simulink model "d_1_dc_motor"  (R2014b)
settings: Solver=ode45  StartTime=0.0  StopTime=10  RelTol=1e-3
values from neighbouring files (symbols this model uses):
  Bm = 0.01    [d_1_dc_motor_parameter.m]    (also in d_2_draw_wt_theta_real.m; d_2_draw_wt_theta_tf.m; d_4_dc_motor_bar_parameter.m; plot.m)
  Jm = 0.000052    (= 5.2e-05)    [d_1_dc_motor_parameter.m]    (also in d_2_draw_wt_theta_real.m; d_2_draw_wt_theta_tf.m; d_4_dc_motor_bar_parameter.m; plot.m)
  Ke = 0.235    [d_1_dc_motor_parameter.m]    (also in d_2_draw_wt_theta_real.m; d_2_draw_wt_theta_tf.m; d_4_dc_motor_bar_parameter.m; plot.m)
  Kt = 0.235    [d_1_dc_motor_parameter.m]    (also in d_2_draw_wt_theta_real.m; d_2_draw_wt_theta_tf.m; d_4_dc_motor_bar_parameter.m; plot.m)
  La = 0.23    [d_1_dc_motor_parameter.m]    (also in d_2_draw_wt_theta_real.m; d_2_draw_wt_theta_tf.m; d_4_dc_motor_bar_parameter.m; plot.m)
  Ra = 2    [d_1_dc_motor_parameter.m]    (also in d_2_draw_wt_theta_real.m; d_2_draw_wt_theta_tf.m; d_4_dc_motor_bar_parameter.m; plot.m)
  Vlimit = 24    [d_1_dc_motor_parameter.m]
libraries: simulink x3
settings Model: Creator=Admin  LastModifiedBy=Admin

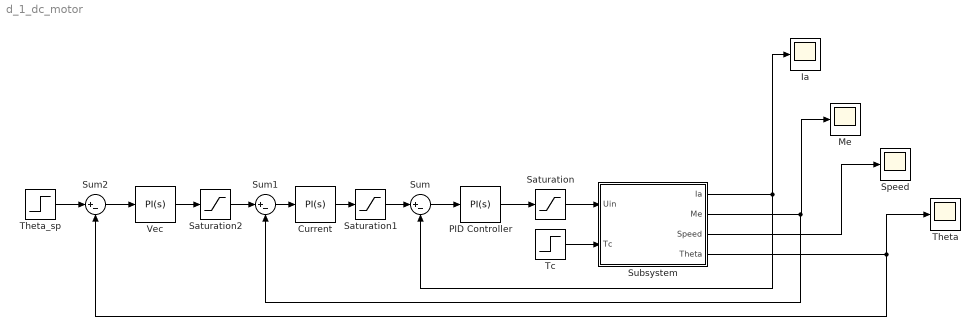
== system d_1_dc_motor ==
  Current : simulink/Continuous/PID Controller  Controller=PI  TimeDomain=Continuous-time  SampleTime=-1  IntegratorMethod=Forward Euler  FilterMethod=Forward Euler  Form=Parallel  P=1  I=1  D=0  N=100  InitialConditionSource=internal  InitialConditionForIntegrator=0  InitialConditionForFilter=0  ExternalReset=none  LimitOutput=off  UpperSaturationLimit=inf  LowerSaturationLimit=-inf  LinearizeAsGain=on  AntiWindupMode=none  Kb=1  TrackingMode=off  Kt=1  PParamMin=[]  PParamMax=[]  IParamMin=[]  IParamMax=[]  DParamMin=[]  DParamMax=[]  NParamMin=[]  NParamMax=[]  KbParamMin=[]  KbParamMax=[]  KtParamMin=[]  KtParamMax=[]  POutMin=[]  POutMax=[]  IOutMin=[]  IOutMax=[]  DOutMin=[]  DOutMax=[]  NOutMin=[]  NOutMax=[]  KbOutMin=[]  KbOutMax=[]  KtOutMin=[]  KtOutMax=[]  IntegratorOutMin=[]  IntegratorOutMax=[]  FilterOutMin=[]  FilterOutMax=[]  SumOutMin=[]  SumOutMax=[]  SumI1OutMin=[]  SumI1OutMax=[]  SumI2OutMin=[]  SumI2OutMax=[]  SumI3OutMin=[]  SumI3OutMax=[]  SumDOutMin=[]  SumDOutMax=[]  SaturationOutMin=[]  SaturationOutMax=[]  IntegratorContinuousStateAttributes=''  IntegratorStateMustResolveToSignalObject=off  IntegratorRTWStateStorageClass=Auto  FilterContinuousStateAttributes=''  FilterStateMustResolveToSignalObject=off  FilterRTWStateStorageClass=Auto  DifferentiatorICPrevScaledInput=0  DifferentiatorOutMin=[]  DifferentiatorOutMax=[]  UseFilter=on
  Ia : Scope
      settings: YMin=0  YMax=10  SaveName=ScopeData2
  Me : Scope
      settings: YMin=-6  YMax=10
  PID Controller : simulink/Continuous/PID Controller  Controller=PI  TimeDomain=Continuous-time  SampleTime=-1  IntegratorMethod=Forward Euler  FilterMethod=Forward Euler  Form=Parallel  P=1  I=1  D=0  N=0  InitialConditionSource=internal  InitialConditionForIntegrator=0  InitialConditionForFilter=0  ExternalReset=none  LimitOutput=off  UpperSaturationLimit=inf  LowerSaturationLimit=-inf  LinearizeAsGain=on  AntiWindupMode=none  Kb=1  TrackingMode=off  Kt=1  PParamMin=[]  PParamMax=[]  IParamMin=[]  IParamMax=[]  DParamMin=[]  DParamMax=[]  NParamMin=[]  NParamMax=[]  KbParamMin=[]  KbParamMax=[]  KtParamMin=[]  KtParamMax=[]  POutMin=[]  POutMax=[]  IOutMin=[]  IOutMax=[]  DOutMin=[]  DOutMax=[]  NOutMin=[]  NOutMax=[]  KbOutMin=[]  KbOutMax=[]  KtOutMin=[]  KtOutMax=[]  IntegratorOutMin=[]  IntegratorOutMax=[]  FilterOutMin=[]  FilterOutMax=[]  SumOutMin=[]  SumOutMax=[]  SumI1OutMin=[]  SumI1OutMax=[]  SumI2OutMin=[]  SumI2OutMax=[]  SumI3OutMin=[]  SumI3OutMax=[]  SumDOutMin=[]  SumDOutMax=[]  SaturationOutMin=[]  SaturationOutMax=[]  IntegratorContinuousStateAttributes=''  IntegratorStateMustResolveToSignalObject=off  IntegratorRTWStateStorageClass=Auto  FilterContinuousStateAttributes=''  FilterStateMustResolveToSignalObject=off  FilterRTWStateStorageClass=Auto  DifferentiatorICPrevScaledInput=0  DifferentiatorOutMin=[]  DifferentiatorOutMax=[]  UseFilter=on
  Saturation : Saturate  UpperLimit=Vlimit  LowerLimit=-Vlimit
  Saturation1 : Saturate  UpperLimit=2  LowerLimit=-2
  Saturation2 : Saturate  UpperLimit=75  LowerLimit=-75
  Speed : Scope
      settings: TimeRange=1.706369139607597  YMin=-34267.66  YMax=-34267.56000000001
  Subsystem : Subsystem
  Sum : Sum  Inputs=|+-
  Sum1 : Sum  Inputs=|+-
  Sum2 : Sum  Inputs=|+-
  Tc : Step  Time=0  After=0  SampleTime=0
  Theta : Scope
      settings: TimeRange=1  YMin=-1  YMax=1  SaveName=ScopeData4
  Theta_sp : Step  Time=0  SampleTime=0
  Vec : simulink/Continuous/PID Controller  Controller=PI  TimeDomain=Continuous-time  SampleTime=-1  IntegratorMethod=Forward Euler  FilterMethod=Forward Euler  Form=Parallel  P=5  I=1  D=0  N=100  InitialConditionSource=internal  InitialConditionForIntegrator=0  InitialConditionForFilter=0  ExternalReset=none  LimitOutput=off  UpperSaturationLimit=inf  LowerSaturationLimit=-inf  LinearizeAsGain=on  AntiWindupMode=none  Kb=1  TrackingMode=off  Kt=1  PParamMin=[]  PParamMax=[]  IParamMin=[]  IParamMax=[]  DParamMin=[]  DParamMax=[]  NParamMin=[]  NParamMax=[]  KbParamMin=[]  KbParamMax=[]  KtParamMin=[]  KtParamMax=[]  POutMin=[]  POutMax=[]  IOutMin=[]  IOutMax=[]  DOutMin=[]  DOutMax=[]  NOutMin=[]  NOutMax=[]  KbOutMin=[]  KbOutMax=[]  KtOutMin=[]  KtOutMax=[]  IntegratorOutMin=[]  IntegratorOutMax=[]  FilterOutMin=[]  FilterOutMax=[]  SumOutMin=[]  SumOutMax=[]  SumI1OutMin=[]  SumI1OutMax=[]  SumI2OutMin=[]  SumI2OutMax=[]  SumI3OutMin=[]  SumI3OutMax=[]  SumDOutMin=[]  SumDOutMax=[]  SaturationOutMin=[]  SaturationOutMax=[]  IntegratorContinuousStateAttributes=''  IntegratorStateMustResolveToSignalObject=off  IntegratorRTWStateStorageClass=Auto  FilterContinuousStateAttributes=''  FilterStateMustResolveToSignalObject=off  FilterRTWStateStorageClass=Auto  DifferentiatorICPrevScaledInput=0  DifferentiatorOutMin=[]  DifferentiatorOutMax=[]  UseFilter=on
  wires:
  Subsystem/1(Ia) -> Ia/1, Sum/2
  Subsystem/2(Me) -> Sum1/2, Me/1
  Subsystem/3(Speed) -> Speed/1
  Subsystem/4(Theta) -> Sum2/2, Theta/1
  Tc/1 -> Subsystem/2(Tc)
  PID Controller/1 -> Saturation/1
  Sum/1 -> PID Controller/1
  Sum1/1 -> Current/1
  Vec/1 -> Saturation2/1
  Sum2/1 -> Vec/1
  Theta_sp/1 -> Sum2/1
  Saturation/1 -> Subsystem/1(Uin)
  Saturation1/1 -> Sum/1
  Current/1 -> Saturation1/1
  Saturation2/1 -> Sum1/1

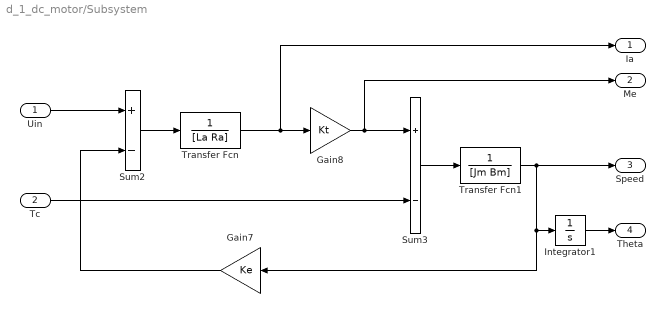
== system d_1_dc_motor/Subsystem ==
  Uin : Inport
  Tc : Inport  Port=2
  Gain7 : Gain  Gain=Ke
  Gain8 : Gain  Gain=Kt
  Integrator1 : Integrator
  Sum2 : Sum  Inputs=+-
  Sum3 : Sum  Inputs=+-
  Transfer Fcn : TransferFcn  Denominator=[La Ra]
  Transfer Fcn1 : TransferFcn  Denominator=[Jm Bm]
  Ia : Outport
  Me : Outport  Port=2
  Speed : Outport  Port=3
  Theta : Outport  Port=4
  wires:
  Gain7/1 -> Sum2/2
  Sum2/1 -> Transfer Fcn/1
  Gain8/1 -> Me/1, Sum3/1
  Transfer Fcn/1 -> Ia/1, Gain8/1
  Uin/1 -> Sum2/1
  Tc/1 -> Sum3/2
  Integrator1/1 -> Theta/1
  Sum3/1 -> Transfer Fcn1/1
  Transfer Fcn1/1 -> Gain7/1, Integrator1/1, Speed/1
